simulink model "decentralized"  (R2023a)
settings: Solver=ode4  StartTime=0.0  StopTime=15  FixedStep=0.001  RelTol=1e-3
values from neighbouring files (symbols this model uses):
  am = [0 1*fmax' 0]    [init.m]
  D_ = distance*W    [init.m]
  g = patch(pp(2,:),pp(1,:),-pp(3,:), v_norm_,'EdgeColor','interp','LineWidth',2)    [demonstration.m]    (also in init.m = 9.8)
  K = K0    [init.m]
  L = D-W    [init.m]
  L0 = ones(n,n)    [init.m]
  M = diag(m)    [init.m]
  m = 11    [demonstration.m]    (also in init.m = [2,1,1,1,1,1,1,1,1,1,1,5]')
  n = n0 + 2    (= 12)    [init.m]
  pp_ = position(:,i)    [demonstration.m]    (also in init.m = [pp_; h0; mass(3)])
  v0 = [zeros(1, 2+2*(n0+2))]'    [init.m]
  W = ones(n,n)    [init.m]

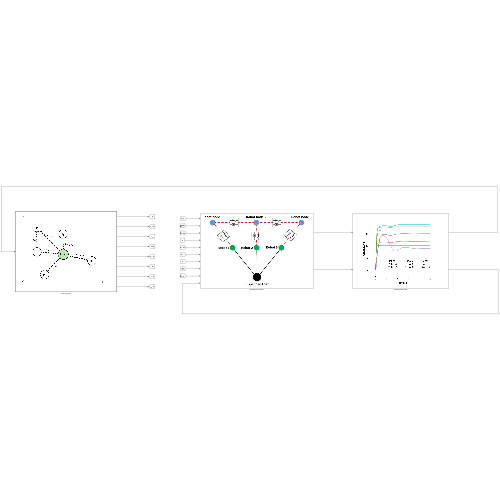
[thumbnail: Simulink's stored preview of the top-level diagram]
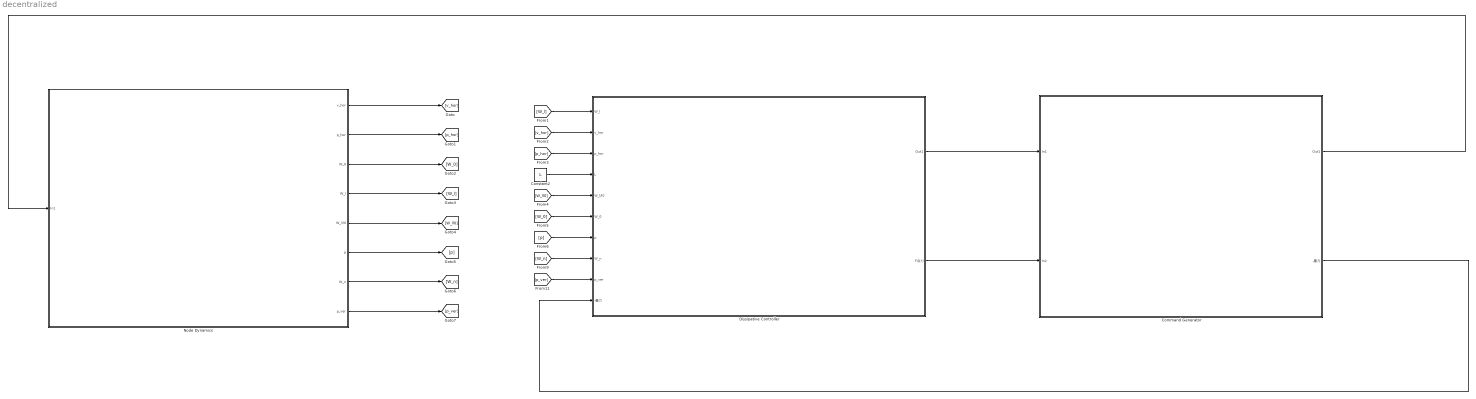
== system decentralized ==
  Command Generator : Subsystem
  Constant2 : Constant  Value=L
  Dissipative Controller : Subsystem
  Node Dynamics : Subsystem
  wires:
  Node Dynamics/1(v_hor) -> [v_hor]
  Node Dynamics/2(p_hor) -> [p_hor]
  Node Dynamics/3(W_0) -> [W_0]
  Node Dynamics/4(W_l) -> [W_l]
  Node Dynamics/5(W_l/l0) -> [W_ll0]
  Node Dynamics/6(p) -> [p]
  Node Dynamics/7(W_n) -> [W_n]
  Node Dynamics/8(p_ver) -> [p_ver]
  [W_l] -> Dissipative Controller/1(W_l)
  [v_hor] -> Dissipative Controller/2(v_hor)
  [p_hor] -> Dissipative Controller/3(p_hor)
  Constant2/1 -> Dissipative Controller/4(L)
  [W_ll0] -> Dissipative Controller/5(W_l/l0)
  [W_0] -> Dissipative Controller/6(W_0)
  [p] -> Dissipative Controller/7(p)
  [W_n] -> Dissipative Controller/8(W_n)
  [p_ver] -> Dissipative Controller/9(p_ver)
  Dissipative Controller/1(Out1) -> Command Generator/1(In1)
  Dissipative Controller/2(F合力) -> Command Generator/2(In2)
  Command Generator/1(Out1) -> Node Dynamics/1(In1)
  Command Generator/2(-重力) -> Dissipative Controller/10(-重力)

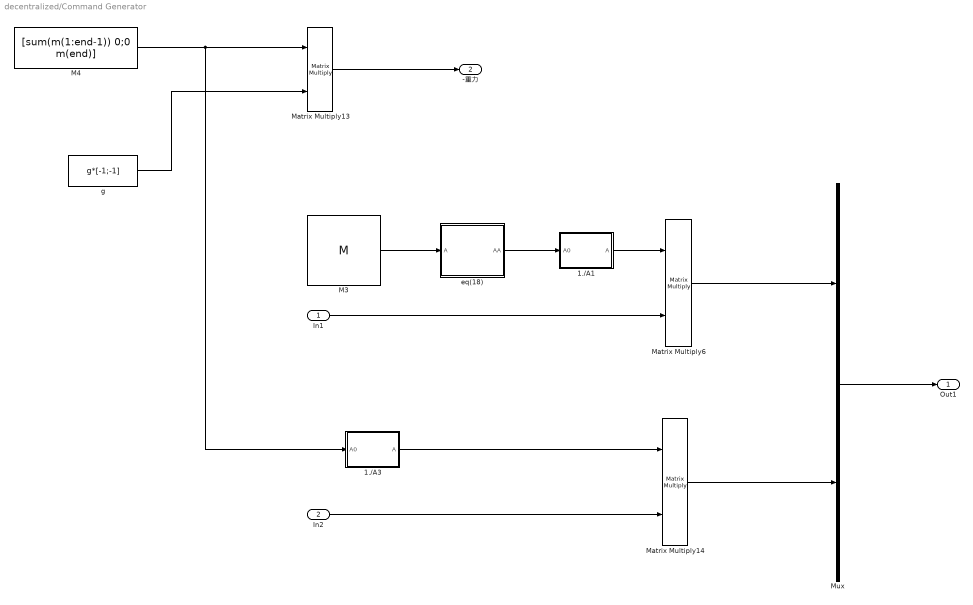
== system decentralized/Command Generator ==
  In1 : Inport
  In2 : Inport  Port=2
  1./A1 : MATLAB Function  TreatAsAtomicUnit=on
  1./A3 : MATLAB Function  TreatAsAtomicUnit=on
  M3 : Constant  Value=M
  M4 : Constant  Value=[sum(m(1:end-1)) 0;0 m(end)]
  Matrix Multiply13 : Product  Multiplication=Matrix(*)
  Matrix Multiply14 : Product  Multiplication=Matrix(*)
  Matrix Multiply6 : Product  Multiplication=Matrix(*)
  Mux : Mux  Inputs=2
  eq(18) : MATLAB Function  TreatAsAtomicUnit=on
  g : Constant  Value=g*[-1;-1]
  Out1 : Outport
  -重力 : Outport  Port=2
  wires:
  g/1 -> Matrix Multiply13/2
  1./A1/1(A) -> Matrix Multiply6/1
  Matrix Multiply14/1 -> Mux/2
  Matrix Multiply13/1 -> -重力/1
  M3/1 -> eq(18)/1(A)
  eq(18)/1(AA) -> 1./A1/1(A0)
  In1/1 -> Matrix Multiply6/2
  1./A3/1(A) -> Matrix Multiply14/1
  Matrix Multiply6/1 -> Mux/1
  M4/1 -> 1./A3/1(A0), Matrix Multiply13/1
  Mux/1 -> Out1/1
  In2/1 -> Matrix Multiply14/2

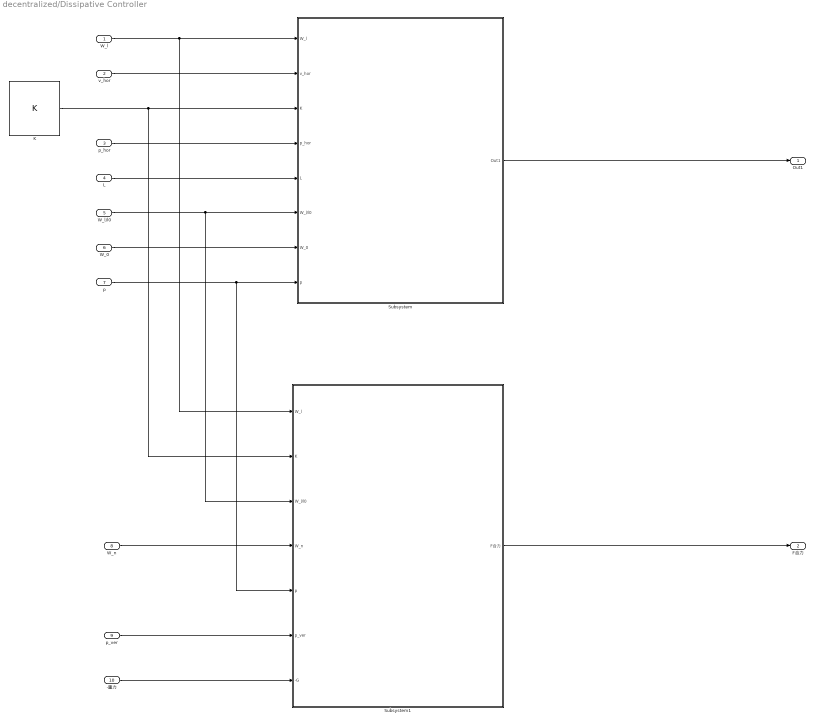
== system decentralized/Dissipative Controller ==
  W_l : Inport
  v_hor : Inport  Port=2
  p_hor : Inport  Port=3
  L : Inport  Port=4
  W_l/l0 : Inport  Port=5
  W_0 : Inport  Port=6
  p : Inport  Port=7
  W_n : Inport  Port=8
  p_ver : Inport  Port=9
  -重力 : Inport  Port=10
  K : Constant  Value=K
  Subsystem : Subsystem
  Subsystem1 : Subsystem
  Out1 : Outport
  F合力 : Outport  Port=2
  wires:
  Subsystem/1(Out1) -> Out1/1
  Subsystem1/1(F合力) -> F合力/1
  K/1 -> Subsystem1/2(K), Subsystem/3(K)
  L/1 -> Subsystem/5(L)
  W_n/1 -> Subsystem1/4(W_n)
  -重力/1 -> Subsystem1/7(-G)
  W_0/1 -> Subsystem/7(W_0)
  p/1 -> Subsystem1/5(p), Subsystem/8(p)
  v_hor/1 -> Subsystem/2(v_hor)
  W_l/1 -> Subsystem/1(W_l), Subsystem1/1(W_l)
  p_ver/1 -> Subsystem1/6(p_ver)
  W_l/l0/1 -> Subsystem/6(W_l/l0), Subsystem1/3(W_l/l0)
  p_hor/1 -> Subsystem/4(p_hor)

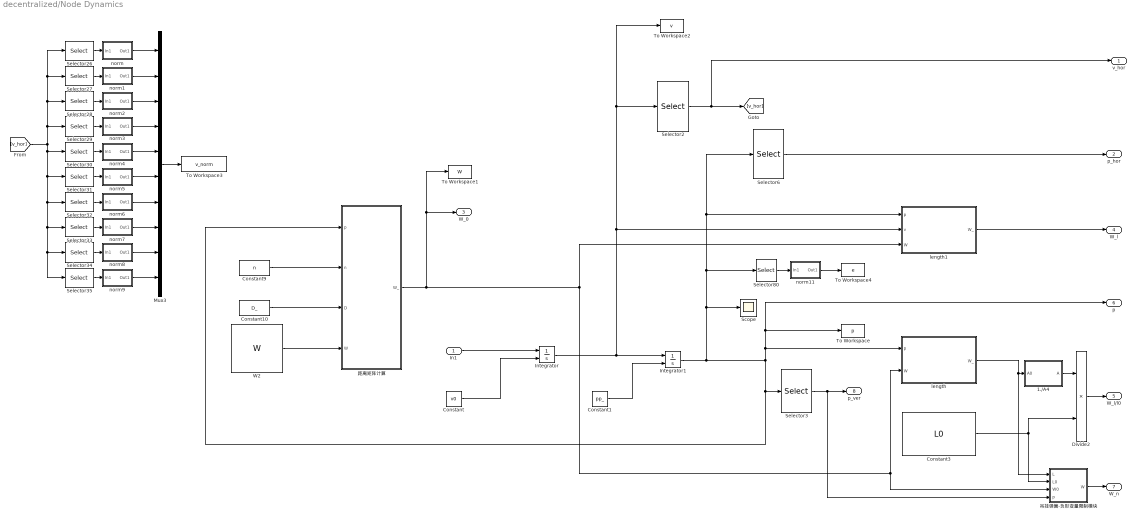
== system decentralized/Node Dynamics ==
  In1 : Inport
  1./A4 : MATLAB Function  TreatAsAtomicUnit=on
  Constant : Constant  Value=v0
  Constant1 : Constant  Value=pp_
  Constant10 : Constant  Value=D_
  Constant3 : Constant  Value=L0
  Constant9 : Constant  Value=n
  Divide2 : Product  Inputs=**
  Integrator : Integrator  InitialConditionSource=external
  Integrator1 : Integrator  InitialConditionSource=external
  Mux3 : Mux  Inputs=10
  Scope : Scope
  Selector2 : Selector  InputPortWidth=2*n+2  IndexOptions=Index vector (dialog)  Indices=[1:2*n]  OutputSizes=1
  Selector26 : Selector  InputPortWidth=2*n  IndexOptions=Index vector (dialog)  Indices=[3,4]  OutputSizes=1
  Selector27 : Selector  InputPortWidth=2*n  IndexOptions=Index vector (dialog)  Indices=[5,6]  OutputSizes=1
  Selector28 : Selector  InputPortWidth=2*n  IndexOptions=Index vector (dialog)  Indices=[7,8]  OutputSizes=1
  Selector29 : Selector  InputPortWidth=2*n  IndexOptions=Index vector (dialog)  Indices=[9,10]  OutputSizes=1
  Selector3 : Selector  InputPortWidth=2*n+2  IndexOptions=Index vector (dialog)  Indices=[2*n+1 2*n+2]  OutputSizes=1
  Selector30 : Selector  InputPortWidth=2*n  IndexOptions=Index vector (dialog)  Indices=[11,12]  OutputSizes=1
  Selector31 : Selector  InputPortWidth=2*n  IndexOptions=Index vector (dialog)  Indices=[13,14]  OutputSizes=1
  Selector32 : Selector  InputPortWidth=2*n  IndexOptions=Index vector (dialog)  Indices=[15,16]  OutputSizes=1
  Selector33 : Selector  InputPortWidth=2*n  IndexOptions=Index vector (dialog)  Indices=[17,18]  OutputSizes=1
  Selector34 : Selector  InputPortWidth=2*n  IndexOptions=Index vector (dialog)  Indices=[19,20]  OutputSizes=1
  Selector35 : Selector  InputPortWidth=2*n  IndexOptions=Index vector (dialog)  Indices=[21,22]  OutputSizes=1
  Selector6 : Selector  InputPortWidth=2*n+2  IndexOptions=Index vector (dialog)  Indices=[1:2*n]  OutputSizes=1
  Selector80 : Selector  InputPortWidth=2*n+2  IndexOptions=Index vector (dialog)  Indices=[2*n,2*n+2]  OutputSizes=1
  To Workspace : ToWorkspace  VariableName=p  SaveFormat=Timeseries  SampleTime=-1
  To Workspace1 : ToWorkspace  VariableName=W  SaveFormat=Timeseries  SampleTime=-1
  To Workspace2 : ToWorkspace  VariableName=v  SaveFormat=Timeseries  SampleTime=-1
  To Workspace3 : ToWorkspace  VariableName=v_norm  SaveFormat=Timeseries  SampleTime=-1
  To Workspace4 : ToWorkspace  VariableName=e  SaveFormat=Timeseries  SampleTime=-1
  W2 : Constant  Value=W
  length : MATLAB Function  TreatAsAtomicUnit=on
  length1 : MATLAB Function  TreatAsAtomicUnit=on
  norm : Subsystem
  norm1 : Subsystem
  norm11 : Subsystem
  norm2 : Subsystem
  norm3 : Subsystem
  norm4 : Subsystem
  norm5 : Subsystem
  norm6 : Subsystem
  norm7 : Subsystem
  norm8 : Subsystem
  norm9 : Subsystem
  吊挂弹簧-负形变量限制模块 : MATLAB Function  TreatAsAtomicUnit=on
  距离矩阵计算 : MATLAB Function  TreatAsAtomicUnit=on
  v_hor : Outport
  p_hor : Outport  Port=2
  W_0 : Outport  Port=3
  W_l : Outport  Port=4
  W_l/l0 : Outport  Port=5
  p : Outport  Port=6
  W_n : Outport  Port=7
  p_ver : Outport  Port=8
  wires:
  Integrator1/1 -> length/1(p), p/1, To Workspace/1, 距离矩阵计算/1(p), Selector3/1, Scope/1, Selector6/1, length1/1(p), Selector80/1
  Selector3/1 -> 吊挂弹簧-负形变量限制模块/4(p), p_ver/1
  Selector6/1 -> p_hor/1
  norm11/1(Out1) -> To Workspace4/1
  In1/1 -> Integrator/1
  length/1(W_) -> 吊挂弹簧-负形变量限制模块/1(L), 1./A4/1(A0)
  Constant10/1 -> 距离矩阵计算/3(D)
  Selector2/1 -> [v_hor], v_hor/1
  Constant/1 -> Integrator/2
  Selector80/1 -> norm11/1(In1)
  length1/1(W_) -> W_l/1
  W2/1 -> 距离矩阵计算/4(W)
  Integrator/1 -> To Workspace2/1, Selector2/1, length1/2(v), Integrator1/1
  1./A4/1(A) -> Divide2/1
  距离矩阵计算/1(W_) -> W_0/1, To Workspace1/1, length1/3(W), 吊挂弹簧-负形变量限制模块/3(W0), length/2(W)
  Constant1/1 -> Integrator1/2
  Constant9/1 -> 距离矩阵计算/2(n)
  Constant3/1 -> 吊挂弹簧-负形变量限制模块/2(L0), Divide2/2
  Divide2/1 -> W_l/l0/1
  吊挂弹簧-负形变量限制模块/1(W) -> W_n/1
  Selector27/1 -> norm1/1(In1)
  Selector31/1 -> norm5/1(In1)
  norm5/1(Out1) -> Mux3/6
  norm/1(Out1) -> Mux3/1
  Mux3/1 -> To Workspace3/1
  norm8/1(Out1) -> Mux3/9
  Selector34/1 -> norm8/1(In1)
  Selector28/1 -> norm2/1(In1)
  Selector30/1 -> norm4/1(In1)
  Selector32/1 -> norm6/1(In1)
  norm1/1(Out1) -> Mux3/2
  Selector33/1 -> norm7/1(In1)
  Selector35/1 -> norm9/1(In1)
  norm4/1(Out1) -> Mux3/5
  Selector29/1 -> norm3/1(In1)
  Selector26/1 -> norm/1(In1)
  norm6/1(Out1) -> Mux3/7
  [v_hor] -> Selector26/1, Selector27/1, Selector28/1, Selector29/1, Selector35/1, Selector34/1, Selector33/1, Selector32/1, Selector31/1, Selector30/1
  norm9/1(Out1) -> Mux3/10
  norm2/1(Out1) -> Mux3/3
  norm3/1(Out1) -> Mux3/4
  norm7/1(Out1) -> Mux3/8

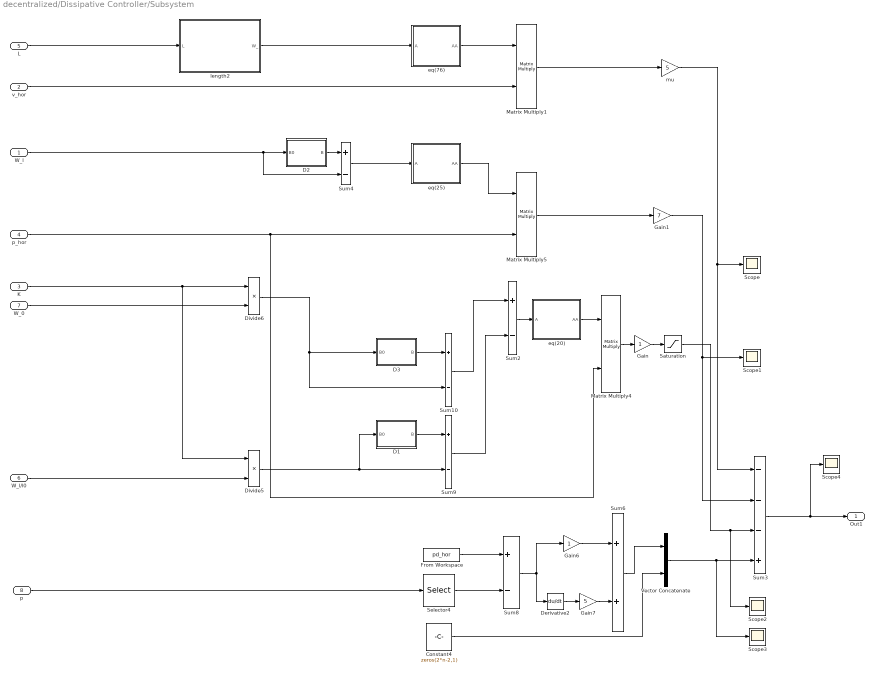
== system decentralized/Dissipative Controller/Subsystem ==
  W_l : Inport
  v_hor : Inport  Port=2
  K : Inport  Port=3
  p_hor : Inport  Port=4
  L : Inport  Port=5
  W_l/l0 : Inport  Port=6
  W_0 : Inport  Port=7
  p : Inport  Port=8
  Constant4 : Constant  Value=zeros(2*n-2,1)
  D1 : MATLAB Function  TreatAsAtomicUnit=on
  D2 : MATLAB Function  TreatAsAtomicUnit=on
  D3 : MATLAB Function  TreatAsAtomicUnit=on
  Derivative2 : Derivative
  Divide5 : Product  Inputs=**
  Divide6 : Product  Inputs=**
  From Workspace : FromWorkspace  VariableName=pd_hor
  Gain : Gain
  Gain1 : Gain  Gain=7
  Gain6 : Gain
  Gain7 : Gain  Gain=5
  Matrix Multiply1 : Product  Multiplication=Matrix(*)
  Matrix Multiply4 : Product  Multiplication=Matrix(*)
  Matrix Multiply5 : Product  Multiplication=Matrix(*)
  Saturation : Saturate  UpperLimit=100  LowerLimit=-100
  Scope{,1..4} (5 alike) : Scope
  Selector4 : Selector  InputPortWidth=2*n+2  IndexOptions=Index vector (dialog)  Indices=[1 2]  OutputSizes=1
  Sum{2,4,8..10} (5 alike) : Sum  Inputs=+-
  Sum3 : Sum  Inputs=---+
  Sum6 : Sum
  Vector Concatenate : Concatenate
  eq(20) : MATLAB Function  TreatAsAtomicUnit=on
  eq(25) : MATLAB Function  TreatAsAtomicUnit=on
  eq(76) : MATLAB Function  TreatAsAtomicUnit=on
  length2 : MATLAB Function  TreatAsAtomicUnit=on
  mu : Gain  Gain=5
  Out1 : Outport
  wires:
  Sum2/1 -> eq(20)/1(A)
  mu/1 -> Scope/1, Sum3/1
  Gain/1 -> Saturation/1
  Gain7/1 -> Sum6/2
  Vector Concatenate/1 -> Scope3/1, Sum3/4
  Sum10/1 -> Sum2/1
  length2/1(W_) -> eq(76)/1(A)
  D1/1(B) -> Sum9/1
  W_0/1 -> Divide6/2
  Sum8/1 -> Gain6/1, Derivative2/1
  Saturation/1 -> Scope2/1, Sum3/3
  Sum9/1 -> Sum2/2
  Sum3/1 -> Scope4/1, Out1/1
  Divide6/1 -> Sum10/2, D3/1(B0)
  eq(20)/1(AA) -> Matrix Multiply4/1
  Selector4/1 -> Sum8/2
  W_l/1 -> D2/1(B0), Sum4/2
  p_hor/1 -> Matrix Multiply4/2, Matrix Multiply5/2
  D2/1(B) -> Sum4/1
  Gain1/1 -> Scope1/1, Sum3/2
  eq(76)/1(AA) -> Matrix Multiply1/1
  L/1 -> length2/1(L)
  Matrix Multiply5/1 -> Gain1/1
  Matrix Multiply4/1 -> Gain/1
  eq(25)/1(AA) -> Matrix Multiply5/1
  p/1 -> Selector4/1
  Divide5/1 -> Sum9/2, D1/1(B0)
  D3/1(B) -> Sum10/1
  Matrix Multiply1/1 -> mu/1
  K/1 -> Divide5/1, Divide6/1
  W_l/l0/1 -> Divide5/2
  Sum6/1 -> Vector Concatenate/1
  From Workspace/1 -> Sum8/1
  Constant4/1 -> Vector Concatenate/2
  Gain6/1 -> Sum6/1
  Derivative2/1 -> Gain7/1
  v_hor/1 -> Matrix Multiply1/2
  Sum4/1 -> eq(25)/1(A)

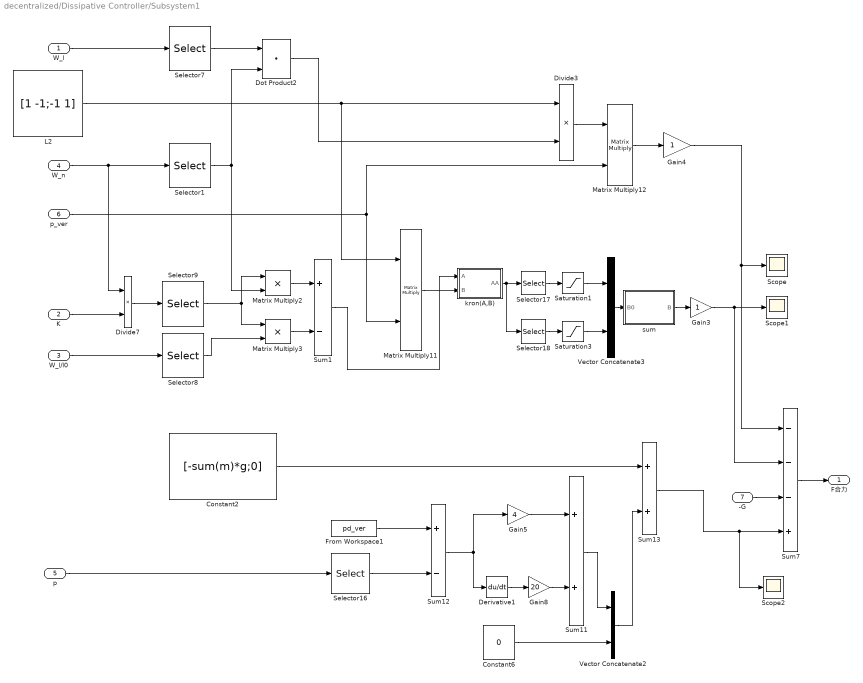
== system decentralized/Dissipative Controller/Subsystem1 ==
  W_l : Inport
  K : Inport  Port=2
  W_l/l0 : Inport  Port=3
  W_n : Inport  Port=4
  p : Inport  Port=5
  p_ver : Inport  Port=6
  -G : Inport  Port=7
  Constant2 : Constant  Value=[-sum(m)*g;0]
  Constant6 : Constant  Value=0
  Derivative1 : Derivative
  Divide3 : Product  Inputs=**
  Divide7 : Product  Inputs=**
  Dot Product2 : DotProduct  OutDataTypeStr=Inherit: Inherit via internal rule
  From Workspace1 : FromWorkspace  VariableName=pd_ver
  Gain3 : Gain
  Gain4 : Gain
  Gain5 : Gain  Gain=4
  Gain8 : Gain  Gain=20
  L2 : Constant  Value=[1 -1;-1 1]
  Matrix Multiply11 : Product  Multiplication=Matrix(*)
  Matrix Multiply12 : Product  Multiplication=Matrix(*)
  Matrix Multiply2 : Product
  Matrix Multiply3 : Product
  Saturation1 : Saturate  UpperLimit=am  LowerLimit=-am
  Saturation3 : Saturate  UpperLimit=am  LowerLimit=-am
  Scope : Scope
  Scope1 : Scope
  Scope2 : Scope
  Selector{1,7..9} (4 alike) : Selector  NumberOfDimensions=2  InputPortWidth=6  IndexOptions=Index vector (dialog),Index vector (dialog)  Indices=n,[1:n]  OutputSizes=1,1
  Selector16 : Selector  InputPortWidth=2*n+2  IndexOptions=Index vector (dialog)  Indices=2*n+1  OutputSizes=1
  Selector17 : Selector  NumberOfDimensions=2  InputPortWidth=6  IndexOptions=Index vector (dialog),Index vector (dialog)  Indices=1,[1:n]  OutputSizes=1,1
  Selector18 : Selector  NumberOfDimensions=2  InputPortWidth=6  IndexOptions=Index vector (dialog),Index vector (dialog)  Indices=2,[1:n]  OutputSizes=1,1
  Sum1 : Sum  Inputs=+-
  Sum11 : Sum
  Sum12 : Sum  Inputs=+-
  Sum13 : Sum
  Sum7 : Sum  Inputs=---+
  Vector Concatenate2 : Concatenate
  Vector Concatenate3 : Concatenate  Mode=Multidimensional array
  kron(A,B) : MATLAB Function  TreatAsAtomicUnit=on
  sum : MATLAB Function  TreatAsAtomicUnit=on
  F合力 : Outport
  wires:
  W_n/1 -> Divide7/1, Selector1/1
  Selector7/1 -> Dot Product2/1
  Sum12/1 -> Gain5/1, Derivative1/1
  Sum1/1 -> kron(A,B)/1(A)
  Vector Concatenate3/1 -> sum/1(B0)
  Gain4/1 -> Scope/1, Sum7/1
  Vector Concatenate2/1 -> Sum13/2
  Matrix Multiply12/1 -> Gain4/1
  -G/1 -> Sum7/3
  kron(A,B)/1(AA) -> Selector17/1, Selector18/1
  K/1 -> Divide7/2
  Selector1/1 -> Matrix Multiply2/2, Dot Product2/2
  Constant2/1 -> Sum13/1
  Constant6/1 -> Vector Concatenate2/2
  W_l/1 -> Selector7/1
  Saturation3/1 -> Vector Concatenate3/2
  Gain8/1 -> Sum11/2
  Sum13/1 -> Scope2/1, Sum7/4
  Matrix Multiply2/1 -> Sum1/1
  Matrix Multiply11/1 -> kron(A,B)/2(B)
  Selector16/1 -> Sum12/2
  Selector9/1 -> Matrix Multiply3/1, Matrix Multiply2/1
  sum/1(B) -> Gain3/1
  Divide3/1 -> Matrix Multiply12/1
  Selector17/1 -> Saturation1/1
  Gain3/1 -> Scope1/1, Sum7/2
  Selector8/1 -> Matrix Multiply3/2
  Gain5/1 -> Sum11/1
  From Workspace1/1 -> Sum12/1
  Divide7/1 -> Selector9/1
  Saturation1/1 -> Vector Concatenate3/1
  L2/1 -> Matrix Multiply11/1, Divide3/1
  Matrix Multiply3/1 -> Sum1/2
  Derivative1/1 -> Gain8/1
  Sum7/1 -> F合力/1
  Selector18/1 -> Saturation3/1
  Sum11/1 -> Vector Concatenate2/1
  p_ver/1 -> Matrix Multiply11/2, Matrix Multiply12/2
  Dot Product2/1 -> Divide3/2
  p/1 -> Selector16/1
  W_l/l0/1 -> Selector8/1

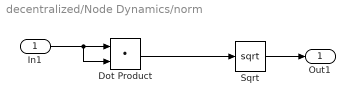
== system decentralized/Node Dynamics/norm ==
  In1 : Inport
  Dot Product : DotProduct  OutDataTypeStr=Inherit: Inherit via internal rule
  Sqrt : Sqrt
  Out1 : Outport
  wires:
  In1/1 -> Dot Product/2, Dot Product/1
  Dot Product/1 -> Sqrt/1
  Sqrt/1 -> Out1/1

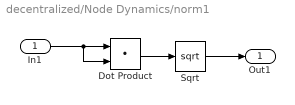
== system decentralized/Node Dynamics/norm1 ==
  In1 : Inport
  Dot Product : DotProduct  OutDataTypeStr=Inherit: Inherit via internal rule
  Sqrt : Sqrt
  Out1 : Outport
  wires:
  Sqrt/1 -> Out1/1
  Dot Product/1 -> Sqrt/1
  In1/1 -> Dot Product/1, Dot Product/2

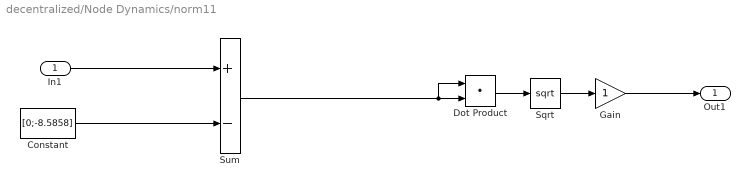
== system decentralized/Node Dynamics/norm11 ==
  In1 : Inport
  Constant : Constant  Value=[0;-8.5858]
  Dot Product : DotProduct  OutDataTypeStr=Inherit: Inherit via internal rule
  Gain : Gain
  Sqrt : Sqrt
  Sum : Sum  Inputs=+-
  Out1 : Outport
  wires:
  Sqrt/1 -> Gain/1
  Dot Product/1 -> Sqrt/1
  Sum/1 -> Dot Product/1, Dot Product/2
  Gain/1 -> Out1/1
  In1/1 -> Sum/1
  Constant/1 -> Sum/2

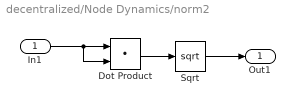
== system decentralized/Node Dynamics/norm2 ==
  In1 : Inport
  Dot Product : DotProduct  OutDataTypeStr=Inherit: Inherit via internal rule
  Sqrt : Sqrt
  Out1 : Outport
  wires:
  In1/1 -> Dot Product/2, Dot Product/1
  Dot Product/1 -> Sqrt/1
  Sqrt/1 -> Out1/1

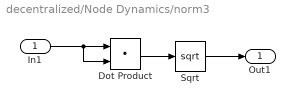
== system decentralized/Node Dynamics/norm3 ==
  In1 : Inport
  Dot Product : DotProduct  OutDataTypeStr=Inherit: Inherit via internal rule
  Sqrt : Sqrt
  Out1 : Outport
  wires:
  Sqrt/1 -> Out1/1
  Dot Product/1 -> Sqrt/1
  In1/1 -> Dot Product/1, Dot Product/2

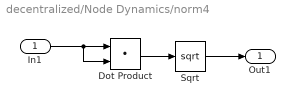
== system decentralized/Node Dynamics/norm4 ==
  In1 : Inport
  Dot Product : DotProduct  OutDataTypeStr=Inherit: Inherit via internal rule
  Sqrt : Sqrt
  Out1 : Outport
  wires:
  In1/1 -> Dot Product/2, Dot Product/1
  Dot Product/1 -> Sqrt/1
  Sqrt/1 -> Out1/1

== system decentralized/Node Dynamics/norm5 ==
  In1 : Inport
  Dot Product : DotProduct  OutDataTypeStr=Inherit: Inherit via internal rule
  Sqrt : Sqrt
  Out1 : Outport
  wires:
  Sqrt/1 -> Out1/1
  Dot Product/1 -> Sqrt/1
  In1/1 -> Dot Product/1, Dot Product/2

== system decentralized/Node Dynamics/norm6 ==
  In1 : Inport
  Dot Product : DotProduct  OutDataTypeStr=Inherit: Inherit via internal rule
  Sqrt : Sqrt
  Out1 : Outport
  wires:
  In1/1 -> Dot Product/2, Dot Product/1
  Dot Product/1 -> Sqrt/1
  Sqrt/1 -> Out1/1

== system decentralized/Node Dynamics/norm7 ==
  In1 : Inport
  Dot Product : DotProduct  OutDataTypeStr=Inherit: Inherit via internal rule
  Sqrt : Sqrt
  Out1 : Outport
  wires:
  Sqrt/1 -> Out1/1
  Dot Product/1 -> Sqrt/1
  In1/1 -> Dot Product/1, Dot Product/2

== system decentralized/Node Dynamics/norm8 ==
  In1 : Inport
  Dot Product : DotProduct  OutDataTypeStr=Inherit: Inherit via internal rule
  Sqrt : Sqrt
  Out1 : Outport
  wires:
  In1/1 -> Dot Product/2, Dot Product/1
  Dot Product/1 -> Sqrt/1
  Sqrt/1 -> Out1/1

== system decentralized/Node Dynamics/norm9 ==
  In1 : Inport
  Dot Product : DotProduct  OutDataTypeStr=Inherit: Inherit via internal rule
  Sqrt : Sqrt
  Out1 : Outport
  wires:
  Sqrt/1 -> Out1/1
  Dot Product/1 -> Sqrt/1
  In1/1 -> Dot Product/1, Dot Product/2

== matlab function decentralized/Node Dynamics/吊挂弹簧-负形变量限制模块 ==
function W = fcn(L,L0,W0,p)
    [m,n] = size(L);
    W = zeros(m,n);
    for i = 1:m
        for j = 1:n
            if i==m || j==n
                if L(i,j)<L0(i,j) || p(1)>p(2) %现长<原长 重物高度比托盘高度高
                    W(i,j) = 0;
                    %W(i,j) = W0(i,j);
                else
                    %W(i,j) = 0;
                    W(i,j) = W0(i,j);
                end
            else 
                    W(i,j) = W0(i,j);
            end
        end
    end
end

== matlab function decentralized/Dissipative Controller/Subsystem/D3 ==
function B = fcn(B0)
[m,n] = size(B0);
B = zeros(m,m);
for i = 1:m
    B(i,i) = sum(B0(i,:)); 
end

== matlab function decentralized/Dissipative Controller/Subsystem1/kron(A,B) ==
function AA = fcn(A,B)
% I = ones(2,1);
AA = kron(A,B);
end

== matlab function decentralized/Dissipative Controller/Subsystem1/sum ==
function B = fcn(B0)
B = sum(B0,2); 
end

== matlab function decentralized/Node Dynamics/距离矩阵计算 ==
function W_ = fcn(p,n,D,W)
%     D = L0(1:n-1, 1:n-1); %感知范围矩阵
% 循环计算两个点之间的距离
    W_ = W;
    for i = 2:n-1
        for j = 2:n-1
            d = norm([p(2*i-1);p(2*i);p(end-1)] - [p(2*j-1);p(2*j);p(end-1)],2);
            if d > D(i,j)
                W_(i,j) = 0;
            end
        end
    end
end

== matlab function decentralized/Node Dynamics/length ==
function W_ = fcn(p,W)
l = size(p,1);
[m,n] = size(W);
W_ = zeros(m,n);
p_ = zeros(3,m);
for kk = 1:m
    if kk == m
        p_(:,kk) = [p(2*kk-1);p(2*kk);p(l)];
    else
        p_(:,kk) = [p(2*kk-1);p(2*kk);p(l-1)];
    end
end
for i = 1:m
    for j = 1:n
        if W(i,j) == 0
            W_(i,j) = 0;
        else
            W_(i,j) = norm((p_(:,i) - p_(:,j)),2);
        end
    end
end

== matlab function decentralized/Dissipative Controller/Subsystem/length2 ==
function W_ = fcn(L)
[m,n] = size(L);
W_ = zeros(m,n);

for i = 1:m
    for j = 1:n
        if i == 1 || j==1
            W_(i,j) = L(i,j);
        else if i==j
            W_(i,j) = 1;
        end
        if i==j & i==m
            W_(i,j) = 0;
        end
        end
    end
end

== matlab function decentralized/Node Dynamics/1.//A4 ==
function A = fcn(A0)
[m,n] = size(A0);
A = zeros(m,n);
for i = 1:m
    for j = 1:n
        if A0(i,j) == 0;
            A(i,j) = 0;
        else
            A(i,j) = 1/A0(i,j);
        end
    end
end

== matlab function decentralized/Command Generator/1.//A1 ==
function A = fcn(A0)
[m,n] = size(A0);
A = zeros(m,n);
for i = 1:m
    for j = i:n
        if A0(i,j) == 0;
            A(i,j) = 0;
        else
            A(i,j) = 1/A0(i,j);
        end
    end
end

== matlab function decentralized/Node Dynamics/length1 ==
function W_ = fcn(p,v,W)
l = size(p,1);
[m,n] = size(W);
W_ = zeros(m,n);
p_ = zeros(3,m);
v_ = zeros(3,m);
for kk = 1:m
    if kk == m
        p_(:,kk) = [p(2*kk-1);p(2*kk);p(l)];
        v_(:,kk) = [v(2*kk-1);v(2*kk);v(l)];
    else
        p_(:,kk) = [p(2*kk-1);p(2*kk);p(l-1)];
        v_(:,kk) = [v(2*kk-1);v(2*kk);v(l-1)];
    end
end

for i = 1:m
    for j = 1:n
        if W(i,j) == 0
            W_(i,j) = 0;
        else
            W_(i,j) = dot((p_(:,i) - p_(:,j)),(v_(:,i) - v_(:,j)))/(norm((p_(:,i) - p_(:,j)),2))^2;
        end
    end
end

== matlab function decentralized/Dissipative Controller/Subsystem/D2 ==
function B = fcn(B0)
[m,n] = size(B0);
B = zeros(m,m);
for i = 1:m
    B(i,i) = sum(B0(i,:)); 
end

== matlab function decentralized/Command Generator/eq(18) ==
function AA = fcn(A)
I = eye(2);
AA = kron(A,I);

== matlab function decentralized/Command Generator/1.//A3 ==
function A = fcn(A0)
[m,n] = size(A0);
A = zeros(m,n);
for i = 1:m
    for j = i:n
        if A0(i,j) == 0;
            A(i,j) = 0;
        else
            A(i,j) = 1/A0(i,j);
        end
    end
end

== matlab function decentralized/Dissipative Controller/Subsystem/eq(20) ==
function AA = fcn(A)
I = eye(2);
AA = kron(A,I);

== matlab function decentralized/Dissipative Controller/Subsystem/eq(25) ==
function AA = fcn(A)
I = eye(2);
AA = kron(A,I);

== matlab function decentralized/Dissipative Controller/Subsystem/D1 ==
function B = fcn(B0)
[m,n] = size(B0);
B = zeros(m,m);
for i = 1:m
    B(i,i) = sum(B0(i,:)); 
end

== matlab function decentralized/Dissipative Controller/Subsystem/eq(76) ==
function AA = fcn(A)
I = eye(2);
AA = kron(A,I);
